simulink model "H036_Separately_excited_DC_motor"  (R2021a)
settings: Solver=VariableStepAuto  StartTime=0.0  StopTime=10.0  RelTol=1e-3
undefined symbols (not defined in the file): K
settings Model: Creator=Pallavi  LastModifiedBy=Pallavi

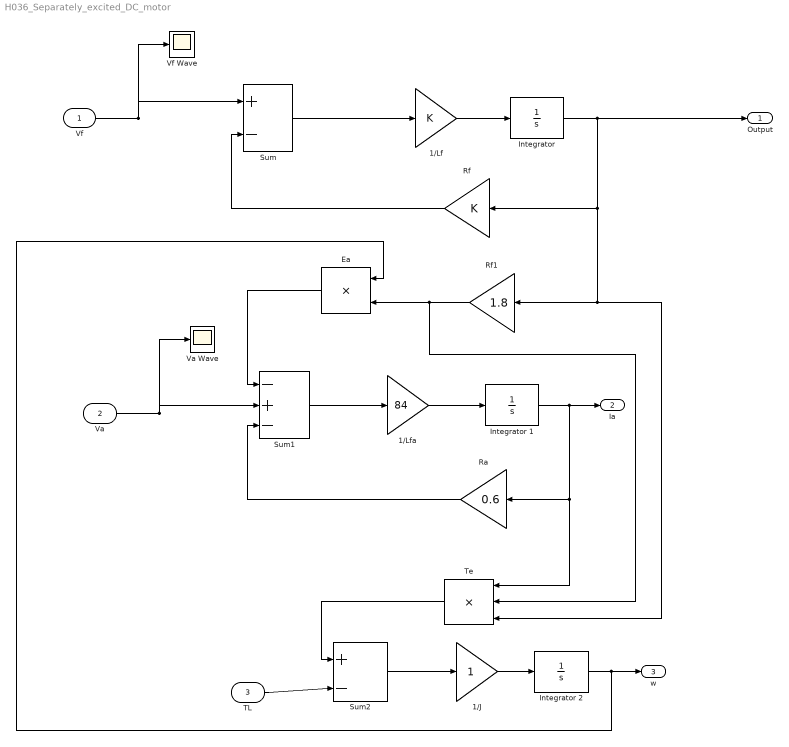
== system H036_Separately_excited_DC_motor ==
  Vf : Inport
  Va : Inport  Port=2
  TL : Inport  Port=3
  1/J : Gain
  1/Lf : Gain  Gain=K
  1/Lfa : Gain  Gain=84
  Ea : Product
  "Integrator " : Integrator
  Integrator 1 : Integrator
  Integrator 2 : Integrator
  Ra : Gain  Gain=0.6
  Rf : Gain  Gain=K
  Rf1 : Gain  Gain=1.8
  Sum : Sum  Inputs=|+-
  Sum1 : Sum  Inputs=|-+-
  Sum2 : Sum  Inputs=|+-
  Te : Product  Inputs=3
  Va Wave : Scope
  Vf Wave : Scope
  Output : Outport
  Ia : Outport  Port=2
  w : Outport  Port=3
  wires:
  Vf/1 -> Vf Wave/1, Sum/1
  Sum/1 -> 1/Lf/1
  1/Lf/1 -> "Integrator "/1
  "Integrator "/1 -> Rf1/1, Te/3, Rf/1, Output/1
  Rf/1 -> Sum/2
  Rf1/1 -> Te/2, Ea/2
  Va/1 -> Sum1/2, Va Wave/1
  Ea/1 -> Sum1/1
  Sum1/1 -> 1/Lfa/1
  1/Lfa/1 -> Integrator 1/1
  Integrator 1/1 -> Te/1, Ra/1, Ia/1
  Ra/1 -> Sum1/3
  Te/1 -> Sum2/1
  TL/1 -> Sum2/2
  Sum2/1 -> 1/J/1
  1/J/1 -> Integrator 2/1
  Integrator 2/1 -> Ea/1, w/1
